simulink model "qp_torq_allocator_base"  (R2024b)
settings: Solver=VariableStepAuto  StartTime=0.0  StopTime=10.0  FixedStep=0.004  RelTol=1e-3
settings Model: Creator=lukec  LastModifiedBy=lukec
settings SolverCC: ZeroCrossControl=DisableAll
settings OptimizationCC: DefaultParameterBehavior=Inlined  EnhancedBackFolding=on  PassReuseOutputArgsAs=Individual arguments  ZeroExternalMemoryAtStartup=off  ZeroInternalMemoryAtStartup=off  OptimizeBlockOrder=speed  DifferentSizesBufferReuse=on  OptimizationCustomize=off  EfficientTunableParamExpr=on
settings DebuggingCC: ParameterTunabilityLossMsg=error
settings HardwareCC: ProdBitPerPointer=32  ProdBitPerSizeT=32  ProdBitPerPtrDiffT=32  ProdLargestAtomicInteger=Long  ProdLargestAtomicFloat=Double  ProdWordSize=32  ProdHWDeviceType=ARM Compatible->ARM Cortex-M
settings SFSimCC: MATLABDynamicMemAlloc=off
settings RTWCC: Description=Embedded Coder  SystemTargetFile=ert.tlc  GenCodeOnly=on  PackageGeneratedCodeAndArtifacts=on  TemplateMakefile=ert_default_tmf  Toolchain=CMake  TargetLang=C++  HalideCodeGeneration=on
settings CodeAppCC: ForceParamTrailComments=on  IgnoreCustomStorageClasses=off  MaxIdLength=255  OperatorAnnotations=on  SimulinkDataObjDesc=on  SFDataObjDesc=on  InsertBlockDesc=on
settings ERTTargetCC: TargetLangStandard=C++17 (ISO)  CodeInterfacePackaging=C++ class  RootIOFormat=Structure reference  ERTCustomFileTemplate=example_file_process.tlc  ArrayContainerType=std::array

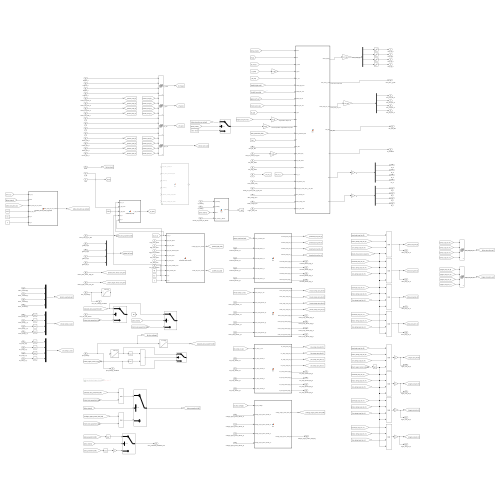
[thumbnail: Simulink's stored preview of the top-level diagram]
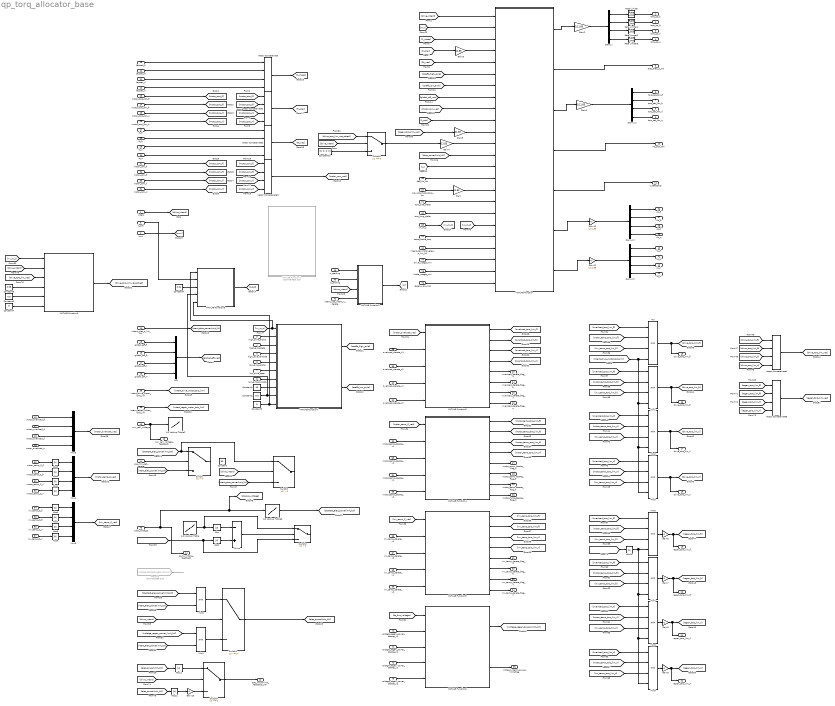
== system qp_torq_allocator_base ==
  intent : Inport
  mux : Inport  Port=2
  high_axle_alpha : Inport  Port=3
  high_axle_beta : Inport  Port=4
  high_axle_lambda : Inport  Port=5
  low_axle_alpha : Inport  Port=6
  low_axle_beta : Inport  Port=7
  low_axle_lambda : Inport  Port=8
  k_opt : Inport  Port=9
  intent_elec_p_lim_kW : Inport  Port=10
  torq_side_delta : Inport  Port=11
  torq_long_delta : Inport  Port=12
  w_starting : Inport  Port=13
  coast_brake_torq : Inport  Port=14
  global_eff_fl : Inport  Port=15
  global_eff_fr : Inport  Port=16
  global_eff_rl : Inport  Port=17
  global_eff_rr : Inport  Port=18
  kappas_fl : Inport  Port=19
  kappas_fr : Inport  Port=20
  kappas_rl : Inport  Port=21
  kappas_rr : Inport  Port=22
  motor_torq_Nm_fl : Inport  Port=23
  motor_torq_Nm_fr : Inport  Port=24
  motor_torq_Nm_rl : Inport  Port=25
  motor_torq_Nm_rr : Inport  Port=26
  fz_fl : Inport  Port=27
  fz_fr : Inport  Port=28
  fz_rl : Inport  Port=29
  fz_rr : Inport  Port=30
  motor_rpm_fl : Inport  Port=31
  motor_rpm_fr : Inport  Port=32
  motor_rpm_rl : Inport  Port=33
  motor_rpm_rr : Inport  Port=34
  vx_m_s : Inport  Port=35
  des_Mz_Nm : Inport  Port=36
  max_tot_motor_torq_Nm : Inport  Port=37
  intent_drive_motor_torq_lim : Inport  Port=38
  intent_regen_motor_torq_lim : Inport  Port=39
  w_ending : Inport  Port=40
  intent_per_motor_elec_p_lim_kW : Inport  Port=41
  intent_use_intent_w_derate : Inport  Port=42  OutDataTypeStr=boolean
  min_cell_voltage : Inport  Port=43
  use_min_cell_derate : Inport  Port=44  OutDataTypeStr=boolean
  pack_voltage : Inport  Port=45
  motor_overload_fl : Inport  Port=46
  motor_overload_fr : Inport  Port=47
  motor_overload_rl : Inport  Port=48
  motor_overload_rr : Inport  Port=49
  motor_temp_C_fl : Inport  Port=50
  motor_temp_C_fr : Inport  Port=51
  motor_temp_C_rl : Inport  Port=52
  motor_temp_C_rr : Inport  Port=53
  inv_temp_C_fl : Inport  Port=54
  inv_temp_C_fr : Inport  Port=55
  inv_temp_C_rl : Inport  Port=56
  inv_temp_C_rr : Inport  Port=57
  overload_derate_x1 : Inport  Port=58
  overload_derate_x2 : Inport  Port=59
  overload_derate_y1 : Inport  Port=60
  overload_derate_y2 : Inport  Port=61
  motor_temp_derate_x1 : Inport  Port=62
  motor_temp_derate_x2 : Inport  Port=63
  motor_temp_derate_y1 : Inport  Port=64
  motor_temp_derate_y2 : Inport  Port=65
  inv_temp_derate_x1 : Inport  Port=66
  inv_temp_derate_x2 : Inport  Port=67
  inv_temp_derate_y1 : Inport  Port=68
  inv_temp_derate_y2 : Inport  Port=69
  voltage_regen_power_derate_x1 : Inport  Port=70
  voltage_regen_power_derate_x2 : Inport  Port=71
  voltage_regen_power_derate_y1 : Inport  Port=72
  voltage_regen_power_derate_y2 : Inport  Port=73
  drive_usage_min : Inport  Port=74
  brake_usage_min : Inport  Port=75
  regen_yaw_max : Inport  Port=76
  1-D Lookup Table : Lookup_n-D  NumberOfTableDimensions=1  BreakpointsForDimension1=[520 530]  Table=[-21 -2]  ExtrapMethod=Clip  UseLastTableValue=on  InternalRulePriority=Speed  RndMeth=Simplest
  1-D Lookup Table2 : Lookup_n-D  NumberOfTableDimensions=1  BreakpointsForDimension1=flip([3.5 3.3 3.15])  Table=flip([78 60 20])  ExtrapMethod=Clip  UseLastTableValue=on  InternalRulePriority=Speed  RndMeth=Simplest
  1-D Lookup Table3 : Lookup_n-D  NumberOfTableDimensions=1  BreakpointsForDimension1=flip([455 445 430])  Table=flip([80 65 40])  ExtrapMethod=Clip  UseLastTableValue=on  InternalRulePriority=Speed  RndMeth=Simplest
  Abs{,1..12} (13 alike) : Abs  SaturateOnIntegerOverflow=off
  Constant : Constant  Value=80
  Constant1 : Constant  Value=40
  Constant10 : Constant  Value=[0; 0; 0; 0]
  Constant2 : Constant  Value=0.5
  Constant3 : Constant  Value=5
  Constant4 : Constant  Value=0.04
  Constant5 : Constant  Value=0.05
  Constant6 : Constant  Value=0.5
  Constant7 : Constant  Value=5
  Demux{,1..3} (4 alike) : Demux
  From10 : From  Commented=on  GotoTag=voltage_derated_regen_torq_lim
  Gain{,3..5} (4 alike) : Gain  Gain=11.83
  Gain{1..2,11..12} (4 alike) : Gain  Gain=1/11.83
  Gain{6..10} (5 alike) : Gain  Gain=-1
  MATLAB Function : MATLAB Function  TreatAsAtomicUnit=on
  MATLAB Function1 : MATLAB Function  Commented=on  TreatAsAtomicUnit=on
  MATLAB Function2 : MATLAB Function  TreatAsAtomicUnit=on
  MATLAB Function3 : MATLAB Function  TreatAsAtomicUnit=on
  MATLAB Function4 : MATLAB Function  TreatAsAtomicUnit=on
  MATLAB Function5 : MATLAB Function  TreatAsAtomicUnit=on
  MATLAB Function6 : MATLAB Function  TreatAsAtomicUnit=on
  MATLAB Function7 : MATLAB Function  TreatAsAtomicUnit=on
  MATLAB Function8 : MATLAB Function  TreatAsAtomicUnit=on
  MATLAB Function9 : MATLAB Function  TreatAsAtomicUnit=on
  Min{,1..3,6..9} (8 alike) : MinMax  Inputs=4
  Min4 : MinMax  Inputs=2
  Min5 : MinMax  Inputs=2
  Minus : Sum  Inputs=-+
  Mux{,3..5} (4 alike) : Mux
  Rate Limiter{,1..3} (4 alike) : RateLimiter  RisingSlewLimit=210  FallingSlewLimit=-210  SampleTimeMode=inherited
  Switch : Switch  Criteria=u2 > Threshold  SaturateOnIntegerOverflow=off  InputSameDT=off
  Switch1 : Switch  Criteria=u2 > Threshold  SaturateOnIntegerOverflow=off  InputSameDT=off
  Switch2 : Switch  Criteria=u2 > Threshold  SaturateOnIntegerOverflow=off  InputSameDT=off
  Switch3 : Switch  SaturateOnIntegerOverflow=off  InputSameDT=off
  Switch4 : Switch  SaturateOnIntegerOverflow=off  InputSameDT=off
  Switch5 : Switch  SaturateOnIntegerOverflow=off  InputSameDT=off
  Vector Concatenate{,1..5} (6 alike) : Concatenate  NumInputs=4  Mode=Multidimensional array
  torq_qp_fl : Outport
  torq_qp_fr : Outport  Port=2
  torq_qp_rl : Outport  Port=3
  torq_qp_rr : Outport  Port=4
  elec_theo_p_kW : Outport  Port=5
  torq_sat_Nm_fl : Outport  Port=6
  torq_sat_Nm_fr : Outport  Port=7
  torq_sat_Nm_rl : Outport  Port=8
  torq_sat_Nm_rr : Outport  Port=9
  Mz_add_Nm : Outport  Port=10
  w_feedback : Outport  Port=11
  elec_powerlimit_feedback_kW : Outport  Port=12
  min_cell_voltage_feedback : Outport  Port=13
  pack_voltage_feedback : Outport  Port=14
  drive_torq_lim_fl : Outport  Port=15
  drive_torq_lim_fr : Outport  Port=16
  drive_torq_lim_rl : Outport  Port=17
  drive_torq_lim_rr : Outport  Port=18
  regen_torq_lim_fl : Outport  Port=19
  regen_torq_lim_fr : Outport  Port=20
  regen_torq_lim_rl : Outport  Port=21
  regen_torq_lim_rr : Outport  Port=22
  overload_derate_flag_fl : Outport  Port=23
  overload_derate_flag_fr : Outport  Port=24
  overload_derate_flag_rl : Outport  Port=25
  overload_derate_flag_rr : Outport  Port=26
  motor_temp_derate_flag_fl : Outport  Port=27
  motor_temp_derate_flag_fr : Outport  Port=28
  motor_temp_derate_flag_rl : Outport  Port=29
  motor_temp_derate_flag_rr : Outport  Port=30
  inv_temp_derate_flag_fl : Outport  Port=31
  inv_temp_derate_flag_fr : Outport  Port=32
  inv_temp_derate_flag_rl : Outport  Port=33
  inv_temp_derate_flag_rr : Outport  Port=34
  voltage_regen_power_limit_flag : Outport  Port=35
  ub_fl : Outport  Port=36
  ub_fr : Outport  Port=37
  ub_rl : Outport  Port=38
  ub_rr : Outport  Port=39
  lb_fl : Outport  Port=40
  lb_fr : Outport  Port=41
  lb_rl : Outport  Port=42
  lb_rr : Outport  Port=43
  wires:
  [Fz_vec] -> MATLAB Function/5(Fz_vec)
  [motor_torq_fl] -> Vector Concatenate1/1
  fz_rl/1 -> Vector Concatenate2/3
  motor_rpm_fl/1 -> [motor_rpm_fl]
  Mux/1 -> [global_eff_vec]
  [motor_torq_rl] -> Vector Concatenate1/3
  Vector Concatenate3/1 -> [motor_rpm_vec]  "rpm_vec"
  Constant10/1 -> Switch3/3
  motor_rpm_rr/1 -> [motor_rpm_rr]
  des_Mz_Nm/1 -> MATLAB Function/15(Mz_des)
  fz_fl/1 -> Vector Concatenate2/1
  low_axle_beta/1 -> MATLAB Function7/6(low_axle_beta)
  Gain5/1 -> MATLAB Function/11("lb ")  "Single Wheel Torque LB"
  fz_rr/1 -> Vector Concatenate2/4
  Gain/1 -> MATLAB Function/16(tot_wheel_torq)
  motor_torq_Nm_rr/1 -> [motor_torq_rr]
  motor_rpm_rl/1 -> [motor_rpm_rl]
  [drive_intent] -> Switch3/2
  MATLAB Function/1(wheel_torque) -> Gain2/1
  MATLAB Function/2(elec_theo_p_kW) -> elec_theo_p_kW/1  "Theo. Elec. Power kW"
  fz_fr/1 -> Vector Concatenate2/2
  [motor_torq_rr] -> Vector Concatenate1/4
  motor_torq_Nm_fr/1 -> [motor_torq_fr]
  [motor_torq_fr] -> Vector Concatenate1/2
  [K_meas] -> MATLAB Function/3(K_meas)
  Vector Concatenate/1 -> [K_meas]  "K_meas"
  high_axle_lambda/1 -> MATLAB Function7/4(high_axle_lambda_base)
  [regen_torq_lim_vec] -> Gain5/1
  global_eff_fl/1 -> Mux/1
  MATLAB Function/3(wheel_torq_sat_vec) -> Gain1/1  "wheel_torq_sat_vec"
  max_tot_motor_torq_Nm/1 -> Gain/1
  Gain4/1 -> MATLAB Function/12("ub ")  "Intent Dependent Single Wheel Torque UB"
  [elec_powerlimit_kW] -> MATLAB Function/13(elec_powerlimit_kW)
  kappas_rr/1 -> Vector Concatenate/4
  intent_elec_p_lim_kW/1 -> [intent_elec_powerlimit_kW]
  high_axle_alpha/1 -> MATLAB Function7/2(high_axle_alpha)
  kappas_fl/1 -> Vector Concatenate/1
  low_axle_alpha/1 -> MATLAB Function7/5(low_axle_alpha)
  torq_side_delta/1 -> MATLAB Function/17(torq_side_delta)
  [drive_torq_lim_vec_sched] -> Switch3/1
  Vector Concatenate2/1 -> [Fz_vec]  "Fz_vec"
  [motor_rpm_fl] -> Vector Concatenate3/1
  kappas_fr/1 -> Vector Concatenate/2
  motor_rpm_fr/1 -> [motor_rpm_fr]
  motor_torq_Nm_rl/1 -> [motor_torq_rl]
  motor_torq_Nm_fl/1 -> [motor_torq_fl]
  [motor_rpm_fr] -> Vector Concatenate3/2
  [motor_rpm_vec] -> MATLAB Function/9(motor_rpm_vec)
  low_axle_lambda/1 -> MATLAB Function7/7(low_axle_lambda_base)
  high_axle_beta/1 -> MATLAB Function7/3(high_axle_beta)
  Gain2/1 -> Demux/1  "motor_torque_qp"
  [coeffs_low_axle] -> MATLAB Function/7(coeffs_low_axle)
  [coeffs_high_axle] -> MATLAB Function/6(coeffs_high_axle)
  [k_opt] -> MATLAB Function/10(K_opt)
  Vector Concatenate1/1 -> [T_prev]  "T_prev"
  [motor_rpm_rl] -> Vector Concatenate3/3
  kappas_rl/1 -> Vector Concatenate/3
  [global_eff_vec] -> MATLAB Function/8(global_eff_vec)
  global_eff_rl/1 -> Mux/3
  coast_brake_torq/1 -> MATLAB Function/20(coast_brake_torq)
  [drive_intent] -> MATLAB Function/1(intent)
  intent/1 -> [drive_intent]
  [motor_rpm_rr] -> Vector Concatenate3/4
  global_eff_fr/1 -> Mux/2
  Gain3/1 -> MATLAB Function/4(T_prev)
  [T_prev] -> Gain3/1
  mux/1 -> [mux]
  global_eff_rr/1 -> Mux/4
  intent_drive_motor_torq_lim/1 -> [intent_drive_motor_torq_lim]
  intent_regen_motor_torq_lim/1 -> [intent_regen_motor_torq_lim]
  torq_long_delta/1 -> MATLAB Function/18(torq_long_delta)
  Gain1/1 -> Demux1/1
  Demux1/1 -> torq_sat_Nm_fl/1
  Demux1/2 -> torq_sat_Nm_fr/1
  Demux1/3 -> torq_sat_Nm_rl/1
  Demux1/4 -> torq_sat_Nm_rr/1
  MATLAB Function/4(Mz_add) -> Mz_add_Nm/1  "Mz_add"
  MATLAB Function/5(w) -> w_feedback/1
  intent_per_motor_elec_p_lim_kW/1 -> MATLAB Function/21(intent_per_motor_elec_p_lim_kW)
  [mux] -> MATLAB Function/2(mux)
  w_starting/1 -> MATLAB Function2/1(w_starting)
  [drive_intent] -> MATLAB Function2/3(intent)
  w_ending/1 -> MATLAB Function2/2(w_ending)
  intent_use_intent_w_derate/1 -> MATLAB Function2/4(use_intent_w_derate)
  MATLAB Function2/1(w_derate) -> [w]
  [w] -> MATLAB Function/14("w ")
  use_min_cell_derate/1 -> Switch/2
  [derated_elec_powerlimit_kW] -> Switch1/1, Switch/1
  [intent_elec_powerlimit_kW] -> Switch/3
  [drive_intent] -> Switch1/2
  [intent_elec_powerlimit_kW] -> Switch1/3
  pack_voltage/1 -> [dc_bus_voltage], 1-D Lookup Table3/1, pack_voltage_feedback/1
  1-D Lookup Table/1 -> Switch2/1, Abs/1
  [intent_regen_motor_torq_lim] -> Switch2/3, Abs1/1
  Abs/1 -> Minus/1
  Abs1/1 -> Minus/2
  Minus/1 -> Switch2/2
  min_cell_voltage/1 -> 1-D Lookup Table2/1, min_cell_voltage_feedback/1
  From10/1 -> ?
  1-D Lookup Table3/1 -> [derated_elec_powerlimit_kW]
  motor_overload_fl/1 -> Mux3/1
  motor_overload_fr/1 -> Mux3/2
  motor_overload_rl/1 -> Mux3/3
  motor_overload_rr/1 -> Mux3/4
  Mux3/1 -> [motor_overload_vec]
  motor_temp_C_fl/1 -> Abs2/1
  motor_temp_C_fr/1 -> Abs3/1
  motor_temp_C_rl/1 -> Abs4/1
  motor_temp_C_rr/1 -> Abs5/1
  Mux4/1 -> [motor_temp_C_vec]
  inv_temp_C_fl/1 -> Abs6/1
  inv_temp_C_fr/1 -> Abs7/1
  inv_temp_C_rl/1 -> Abs8/1
  inv_temp_C_rr/1 -> Abs9/1
  Mux5/1 -> [inv_temp_C_vec]
  [motor_overload_vec] -> MATLAB Function3/1(motor_overload_vec)
  overload_derate_x1/1 -> MATLAB Function3/2(overload_derate_x1)
  overload_derate_x2/1 -> MATLAB Function3/3(overload_derate_x2)
  overload_derate_y1/1 -> MATLAB Function3/4(overload_derate_y1)
  overload_derate_y2/1 -> MATLAB Function3/5(overload_derate_y2)
  [motor_temp_C_vec] -> MATLAB Function4/1(motor_temp_C_vec)
  motor_temp_derate_x1/1 -> MATLAB Function4/2(motor_temp_derate_x1)
  motor_temp_derate_x2/1 -> MATLAB Function4/3(motor_temp_derate_x2)
  motor_temp_derate_y1/1 -> MATLAB Function4/4(motor_temp_derate_y1)
  motor_temp_derate_y2/1 -> MATLAB Function4/5(motor_temp_derate_y2)
  Abs2/1 -> Mux4/1
  Abs3/1 -> Mux4/2
  Abs4/1 -> Mux4/3
  Abs5/1 -> Mux4/4
  Abs6/1 -> Mux5/1
  Abs7/1 -> Mux5/2
  Abs8/1 -> Mux5/3
  Abs9/1 -> Mux5/4
  [inv_temp_C_vec] -> MATLAB Function5/1(inv_temp_C_vec)
  inv_temp_derate_x1/1 -> MATLAB Function5/2(inv_temp_derate_x1)
  inv_temp_derate_x2/1 -> MATLAB Function5/3(inv_temp_derate_x2)
  inv_temp_derate_y1/1 -> MATLAB Function5/4(inv_temp_derate_y1)
  inv_temp_derate_y2/1 -> MATLAB Function5/5(inv_temp_derate_y2)
  MATLAB Function3/1(overload_torq_lim_fl) -> [overload_torq_lim_fl]
  MATLAB Function3/2(overload_torq_lim_fr) -> [overload_torq_lim_fr]
  MATLAB Function3/3(overload_torq_lim_rl) -> [overload_torq_lim_rl]
  MATLAB Function3/4(overload_torq_lim_rr) -> [overload_torq_lim_rr]
  MATLAB Function4/1(motor_temp_torq_lim_fl) -> [motor_temp_torq_lim_fl]
  MATLAB Function4/2(motor_temp_torq_lim_fr) -> [motor_temp_torq_lim_fr]
  MATLAB Function4/3(motor_temp_torq_lim_rl) -> [motor_temp_torq_lim_rl]
  MATLAB Function4/4(motor_temp_torq_lim_rr) -> [motor_temp_torq_lim_rr]
  MATLAB Function5/1(inv_temp_torq_lim_fl) -> [inv_temp_torq_lim_fl]
  MATLAB Function5/2(inv_temp_torq_lim_fr) -> [inv_temp_torq_lim_fr]
  MATLAB Function5/3(inv_temp_torq_lim_rl) -> [inv_temp_torq_lim_rl]
  MATLAB Function5/4(inv_temp_torq_lim_rr) -> [inv_temp_torq_lim_rr]
  [motor_temp_torq_lim_fl] -> Min/2
  [inv_temp_torq_lim_fl] -> Min/3
  [overload_torq_lim_fl] -> Min/1
  [overload_torq_lim_fr] -> Min1/1
  [inv_temp_torq_lim_fr] -> Min1/3
  [motor_temp_torq_lim_fr] -> Min1/2
  [motor_temp_torq_lim_rr] -> Min3/2
  [inv_temp_torq_lim_rr] -> Min3/3
  [overload_torq_lim_rr] -> Min3/1
  [overload_torq_lim_rl] -> Min2/1
  [inv_temp_torq_lim_rl] -> Min2/3
  [motor_temp_torq_lim_rl] -> Min2/2
  Min/1 -> drive_torq_lim_fl/1, [drive_torq_lim_fl]
  Min1/1 -> drive_torq_lim_fr/1, [drive_torq_lim_fr]
  Min2/1 -> drive_torq_lim_rl/1, [drive_torq_lim_rl]
  Min3/1 -> drive_torq_lim_rr/1, [drive_torq_lim_rr]
  [intent_drive_motor_torq_lim] -> Min2/4, Min3/4, Min1/4, Min/4
  [drive_torq_lim_fl] -> Vector Concatenate4/1
  [drive_torq_lim_fr] -> Vector Concatenate4/2
  [drive_torq_lim_rl] -> Vector Concatenate4/3
  [drive_torq_lim_rr] -> Vector Concatenate4/4
  Vector Concatenate4/1 -> [drive_torq_lim_vec]  "drive_torq_lim_vec"
  [dc_bus_voltage] -> MATLAB Function6/1(dc_bus_voltage)
  voltage_regen_power_derate_x1/1 -> MATLAB Function6/2(voltage_regen_power_derate_x1)
  voltage_regen_power_derate_x2/1 -> MATLAB Function6/3(voltage_regen_power_derate_x2)
  voltage_regen_power_derate_y1/1 -> MATLAB Function6/4(voltage_regen_power_derate_y1)
  voltage_regen_power_derate_y2/1 -> MATLAB Function6/5(voltage_regen_power_derate_y2)
  MATLAB Function6/1(voltage_regen_power_limit_kW) -> [voltage_regen_power_limit_kW]
  [drive_intent] -> Switch4/2
  [voltage_regen_power_limit_kW] -> Min4/1
  [intent_elec_powerlimit_kW] -> Min4/2
  [derated_elec_powerlimit_kW] -> Min5/1
  [intent_elec_powerlimit_kW] -> Min5/2
  Min5/1 -> Switch4/1
  Min4/1 -> Switch4/3
  Switch4/1 -> [elec_powerlimit_kW]
  [intent_regen_motor_torq_lim] -> Abs10/1
  Min9/1 -> Gain9/1
  Min8/1 -> Gain8/1
  Min7/1 -> Gain7/1
  Min6/1 -> Gain6/1
  [motor_temp_torq_lim_rl] -> Min8/2
  [inv_temp_torq_lim_rl] -> Min8/3
  [overload_torq_lim_rl] -> Min8/1
  [overload_torq_lim_rr] -> Min9/1
  [inv_temp_torq_lim_rr] -> Min9/3
  [motor_temp_torq_lim_rr] -> Min9/2
  [motor_temp_torq_lim_fr] -> Min7/2
  [inv_temp_torq_lim_fr] -> Min7/3
  [overload_torq_lim_fr] -> Min7/1
  [overload_torq_lim_fl] -> Min6/1
  [inv_temp_torq_lim_fl] -> Min6/3
  [motor_temp_torq_lim_fl] -> Min6/2
  Abs10/1 -> Min6/4, Min7/4, Min9/4, Min8/4
  Gain6/1 -> regen_torq_lim_fl/1, [regen_torq_lim_fl]
  Gain7/1 -> regen_torq_lim_fr/1, [regen_torq_lim_fr]
  Gain8/1 -> regen_torq_lim_rl/1, [regen_torq_lim_rl]
  Gain9/1 -> regen_torq_lim_rr/1, [regen_torq_lim_rr]
  Vector Concatenate5/1 -> [regen_torq_lim_vec]  "regen_torq_lim_vec"
  [regen_torq_lim_rr] -> Vector Concatenate5/4
  [regen_torq_lim_rl] -> Vector Concatenate5/3
  [regen_torq_lim_fr] -> Vector Concatenate5/2
  [regen_torq_lim_fl] -> Vector Concatenate5/1
  MATLAB Function3/5(overload_derate_flag_fl) -> overload_derate_flag_fl/1
  MATLAB Function3/6(overload_derate_flag_fr) -> overload_derate_flag_fr/1
  MATLAB Function3/7(overload_derate_flag_rl) -> overload_derate_flag_rl/1
  MATLAB Function3/8(overload_derate_flag_rr) -> overload_derate_flag_rr/1
  MATLAB Function4/5(motor_temp_derate_flag_fl) -> motor_temp_derate_flag_fl/1
  MATLAB Function4/6(motor_temp_derate_flag_fr) -> motor_temp_derate_flag_fr/1
  MATLAB Function4/7(motor_temp_derate_flag_rl) -> motor_temp_derate_flag_rl/1
  MATLAB Function4/8(motor_temp_derate_flag_rr) -> motor_temp_derate_flag_rr/1
  MATLAB Function5/5(inv_temp_derate_flag_fl) -> inv_temp_derate_flag_fl/1
  MATLAB Function5/6(inv_temp_derate_flag_fr) -> inv_temp_derate_flag_fr/1
  MATLAB Function5/7(inv_temp_derate_flag_rl) -> inv_temp_derate_flag_rl/1
  MATLAB Function5/8(inv_temp_derate_flag_rr) -> inv_temp_derate_flag_rr/1
  MATLAB Function6/2(voltage_regen_power_limit_flag) -> voltage_regen_power_limit_flag/1
  [drive_intent] -> Switch5/2
  [elec_powerlimit_kW] -> Abs11/1
  [elec_powerlimit_kW] -> Abs12/1
  Abs11/1 -> Switch5/1
  Abs12/1 -> Gain10/1
  Gain10/1 -> Switch5/3
  Switch5/1 -> elec_powerlimit_feedback_kW/1
  Switch3/1 -> Gain4/1
  MATLAB Function/7(lb) -> Gain11/1
  MATLAB Function/6(ub) -> Gain12/1
  Gain12/1 -> Demux2/1  "ub"
  Demux2/1 -> ub_fl/1
  Demux2/2 -> ub_fr/1
  Demux2/3 -> ub_rl/1
  Demux2/4 -> ub_rr/1
  Demux3/4 -> lb_rr/1
  Demux3/3 -> lb_rl/1
  Demux3/2 -> lb_fr/1
  Gain11/1 -> Demux3/1  "ub"
  Demux3/1 -> lb_fl/1
  drive_usage_min/1 -> MATLAB Function/22(drive_usage_min)
  brake_usage_min/1 -> MATLAB Function/23(brake_usage_min)
  Demux/1 -> Rate Limiter/1
  Demux/2 -> Rate Limiter1/1
  Demux/3 -> Rate Limiter2/1
  Demux/4 -> Rate Limiter3/1
  Rate Limiter/1 -> torq_qp_fl/1
  Rate Limiter1/1 -> torq_qp_fr/1
  Rate Limiter2/1 -> torq_qp_rl/1
  Rate Limiter3/1 -> torq_qp_rr/1
  vx_m_s/1 -> [vx_m_s]
  [vx_m_s] -> MATLAB Function/19(vx_m_s)
  [vx_m_s] -> MATLAB Function8/1(vx_m_s), MATLAB Function7/1(vx_m_s)
  Constant1/1 -> MATLAB Function7/8(delta_lambda_low)
  Constant2/1 -> MATLAB Function8/4(vx_lo), MATLAB Function7/9(vx_lo)
  Constant3/1 -> MATLAB Function8/5(vx_hi), MATLAB Function7/10(vx_hi)
  MATLAB Function7/1(coeffs_high_axle_sched) -> [coeffs_high_axle]
  MATLAB Function7/2(coeffs_low_axle_sched) -> [coeffs_low_axle]
  Constant4/1 -> MATLAB Function8/3(k_opt_low)
  k_opt/1 -> MATLAB Function8/2(k_opt_nom)
  MATLAB Function8/1(k_opt_sched) -> [k_opt]
  [drive_torq_lim_vec] -> MATLAB Function9/3(drive_torq_lim_vec_base)
  Constant5/1 -> MATLAB Function9/4(low_cap_min)
  Constant6/1 -> MATLAB Function9/5(vx_lo)
  Constant7/1 -> MATLAB Function9/6(vx_hi)
  [drive_intent] -> MATLAB Function9/2(intent)
  [vx_m_s] -> MATLAB Function9/1(vx_m_s)
  MATLAB Function9/1(drive_torq_lim_vec_sched) -> [drive_torq_lim_vec_sched]
  regen_yaw_max/1 -> MATLAB Function/24(regen_yaw_max)

== matlab function qp_torq_allocator_base/MATLAB Function4 ==
  data: motor_temp_C_vec input; motor_temp_torq_lim_fl output; motor_temp_derate_x1 input; motor_temp_derate_x2 input; motor_temp_derate_y1 input; motor_temp_derate_y2 input; motor_temp_torq_lim_fr output; motor_temp_torq_lim_rl output; motor_temp_torq_lim_rr output; motor_temp_derate_flag_fl output; motor_temp_derate_flag_fr output; motor_temp_derate_flag_rl output; motor_temp_derate_flag_rr output
function  [motor_temp_torq_lim_fl, motor_temp_torq_lim_fr, motor_temp_torq_lim_rl, motor_temp_torq_lim_rr, motor_temp_derate_flag_fl, motor_temp_derate_flag_fr, motor_temp_derate_flag_rl, motor_temp_derate_flag_rr] = fcn(motor_temp_C_vec, motor_temp_derate_x1, motor_temp_derate_x2, motor_temp_derate_y1, motor_temp_derate_y2)

overload_torq_lim = zeros(4, 1);
overload_derate_flag = zeros(4, 1);

for i = 1:length(motor_temp_C_vec)
    if motor_temp_C_vec(i) > motor_temp_derate_x2
        motor_temp_C_vec(i) = motor_temp_derate_x2;
    end

    if motor_temp_C_vec(i) < motor_temp_derate_x1
        motor_temp_C_vec(i) = motor_temp_derate_x1;
    end

    overload_torq_lim(i) = interp1([motor_temp_derate_x1, motor_temp_derate_x2], [motor_temp_derate_y1, motor_temp_derate_y2], motor_temp_C_vec(i));
    
    if overload_torq_lim(i) < motor_temp_derate_y1
        overload_derate_flag(i) = 1;
    end
end

motor_temp_torq_lim_fl = overload_torq_lim(1);
motor_temp_torq_lim_fr = overload_torq_lim(2);
motor_temp_torq_lim_rl = overload_torq_lim(3);
motor_temp_torq_lim_rr = overload_torq_lim(4);

motor_temp_derate_flag_fl = overload_derate_flag(1);
motor_temp_derate_flag_fr = overload_derate_flag(2);
motor_temp_derate_flag_rl = overload_derate_flag(3);
motor_temp_derate_flag_rr = overload_derate_flag(4);

== matlab function qp_torq_allocator_base/MATLAB Function5 ==
  data: inv_temp_C_vec input; inv_temp_torq_lim_fl output; inv_temp_derate_x1 input; inv_temp_derate_x2 input; inv_temp_derate_y1 input; inv_temp_derate_y2 input; inv_temp_torq_lim_fr output; inv_temp_torq_lim_rl output; inv_temp_torq_lim_rr output; inv_temp_derate_flag_fl output; inv_temp_derate_flag_fr output; inv_temp_derate_flag_rl output; inv_temp_derate_flag_rr output
function  [inv_temp_torq_lim_fl, inv_temp_torq_lim_fr, inv_temp_torq_lim_rl, inv_temp_torq_lim_rr, inv_temp_derate_flag_fl, inv_temp_derate_flag_fr, inv_temp_derate_flag_rl, inv_temp_derate_flag_rr] = fcn(inv_temp_C_vec, inv_temp_derate_x1, inv_temp_derate_x2, inv_temp_derate_y1, inv_temp_derate_y2)

overload_torq_lim = zeros(4, 1);
overload_derate_flag = zeros(4, 1);

for i = 1:length(inv_temp_C_vec)
    if inv_temp_C_vec(i) > inv_temp_derate_x2
        inv_temp_C_vec(i) = inv_temp_derate_x2;
    end

    if inv_temp_C_vec(i) < inv_temp_derate_x1
        inv_temp_C_vec(i) = inv_temp_derate_x1;
    end

    overload_torq_lim(i) = interp1([inv_temp_derate_x1, inv_temp_derate_x2], [inv_temp_derate_y1, inv_temp_derate_y2], inv_temp_C_vec(i));
    
    if overload_torq_lim(i) < inv_temp_derate_y1
        overload_derate_flag(i) = 1;
    end
end

inv_temp_torq_lim_fl = overload_torq_lim(1);
inv_temp_torq_lim_fr = overload_torq_lim(2);
inv_temp_torq_lim_rl = overload_torq_lim(3);
inv_temp_torq_lim_rr = overload_torq_lim(4);

inv_temp_derate_flag_fl = overload_derate_flag(1);
inv_temp_derate_flag_fr = overload_derate_flag(2);
inv_temp_derate_flag_rl = overload_derate_flag(3);
inv_temp_derate_flag_rr = overload_derate_flag(4);

== matlab function qp_torq_allocator_base/MATLAB Function6 ==
  data: dc_bus_voltage input; voltage_regen_power_limit_kW output; voltage_regen_power_derate_x1 input; voltage_regen_power_derate_x2 input; voltage_regen_power_derate_y1 input; voltage_regen_power_derate_y2 input; voltage_regen_power_limit_flag output
function [voltage_regen_power_limit_kW, voltage_regen_power_limit_flag] = fcn(dc_bus_voltage, voltage_regen_power_derate_x1, voltage_regen_power_derate_x2, voltage_regen_power_derate_y1, voltage_regen_power_derate_y2)

voltage_regen_power_limit_flag = 0;

if dc_bus_voltage < voltage_regen_power_derate_x1
    dc_bus_voltage = voltage_regen_power_derate_x1;
end

if dc_bus_voltage > voltage_regen_power_derate_x2
    dc_bus_voltage = voltage_regen_power_derate_x2;
end

voltage_regen_power_limit_kW = interp1([voltage_regen_power_derate_x1, voltage_regen_power_derate_x2], [voltage_regen_power_derate_y1, voltage_regen_power_derate_y2], dc_bus_voltage);


if voltage_regen_power_limit_kW < voltage_regen_power_derate_y1
    voltage_regen_power_limit_flag = 1;
end

== matlab function qp_torq_allocator_base/MATLAB Function7 ==
  data: vx_m_s input; coeffs_high_axle_sched output; high_axle_alpha input; high_axle_beta input; high_axle_lambda_base input; low_axle_alpha input; low_axle_beta input; low_axle_lambda_base input; delta_lambda_low input; vx_lo input; vx_hi input; coeffs_low_axle_sched output
function [coeffs_high_axle_sched, coeffs_low_axle_sched] = ...
    schedule_axle_coeffs(vx_m_s, ...
    high_axle_alpha, high_axle_beta, high_axle_lambda_base, ...
    low_axle_alpha,  low_axle_beta,  low_axle_lambda_base, ...
    delta_lambda_low, vx_lo, vx_hi)

    s_vx = (vx_m_s - vx_lo) / (vx_hi - vx_lo);
    s_vx = min(max(s_vx, 0), 1);

    lambda_high_sched = high_axle_lambda_base;
    lambda_low_sched  = low_axle_lambda_base + (1 - s_vx) * delta_lambda_low;

    coeffs_high_axle_sched = [high_axle_alpha; high_axle_beta; lambda_high_sched];
    coeffs_low_axle_sched  = [low_axle_alpha;  low_axle_beta;  lambda_low_sched];
end

== matlab function qp_torq_allocator_base/MATLAB Function8 ==
  data: vx_m_s input; k_opt_sched output; k_opt_nom input; k_opt_low input; vx_lo input; vx_hi input
function k_opt_sched = schedule_kopt(vx_m_s, k_opt_nom, k_opt_low, vx_lo, vx_hi)

    s_vx = (vx_m_s - vx_lo) / (vx_hi - vx_lo);
    s_vx = min(max(s_vx, 0), 1);

    k_opt_sched = k_opt_low + s_vx * (k_opt_nom - k_opt_low);
end

== matlab function qp_torq_allocator_base/MATLAB Function9 ==
  data: vx_m_s input; drive_torq_lim_vec_sched output; intent input; drive_torq_lim_vec_base input; low_cap_min input; vx_lo input; vx_hi input
function drive_torq_lim_vec_sched = schedule_drive_limits_highlow( ...
    vx_m_s, intent, drive_torq_lim_vec_base, low_cap_min, vx_lo, vx_hi)

    s_vx = (vx_m_s - vx_lo) / (vx_hi - vx_lo);
    s_vx = min(max(s_vx, 0), 1);

    gamma_low = low_cap_min + (1 - low_cap_min) * s_vx;

    drive_torq_lim_vec_sched = drive_torq_lim_vec_base;

    if intent >= 0
        % accel/coast: low axle = front = FL, FR
        drive_torq_lim_vec_sched(1) = gamma_low * drive_torq_lim_vec_base(1);
        drive_torq_lim_vec_sched(2) = gamma_low * drive_torq_lim_vec_base(2);
    else
        % braking: low axle = rear = RL, RR
        drive_torq_lim_vec_sched(3) = gamma_low * drive_torq_lim_vec_base(3);
        drive_torq_lim_vec_sched(4) = gamma_low * drive_torq_lim_vec_base(4);
    end
end

== matlab function qp_torq_allocator_base/MATLAB Function ==
  data: intent input; mux input; K_meas input; wheel_torque output; T_prev input; Fz_vec input; coeffs_high_axle input; coeffs_low_axle input; global_eff_vec input; motor_rpm_vec input; K_opt input; lb input; ub input; elec_theo_p_kW output; wheel_torq_sat_vec output; elec_powerlimit_kW input; w input; Mz_des input; tot_wheel_torq input; Mz_add output; torq_side_delta input; torq_long_delta input; vx_m_s input; coast_brake_torq input; w output; ub output; intent_per_motor_elec_p_lim_kW input; lb output; drive_usage_min input; brake_usage_min input; regen_yaw_max input
function [wheel_torque, elec_theo_p_kW, wheel_torq_sat_vec, Mz_add, w, ub, lb] = fcn(intent, mux, K_meas, T_prev, Fz_vec, ...
    coeffs_high_axle, coeffs_low_axle, global_eff_vec, motor_rpm_vec, K_opt, lb, ub, elec_powerlimit_kW, w, Mz_des, tot_wheel_torq, ...
    torq_side_delta, torq_long_delta, vx_m_s, coast_brake_torq, intent_per_motor_elec_p_lim_kW, drive_usage_min, brake_usage_min, regen_yaw_max)

    % if w < 0.08
    %     w = 0.08;
    % end

    % drive_usage_bias = 0.8;
    % brake_usage_bias = 0.9;

    % =========================================================================
    % Constants / geometry
    % =========================================================================
    tot_wheel_torq = abs(tot_wheel_torq);

    rpm2rad_s = 0.10472;
    r  = 0.2;       % effective tire radius, an approximation [m]
    ht = 1.2 / 2;   % half-track [m]

    % =========================================================================
    % Interpolation data for longitudinal stiffness approximation C_kappa(Fz)
    % =========================================================================
    Fz_testpoints = [-100	-150	-200	-250	-300	-350	-400	-450	-500	-550	-600	-650	-700	-750	-800	-850	-900	-950	-1000	-1050	-1100	-1150	-1200	-1250	-1300	-1350	-1400	-1450	-1500	-1550	-1600	-1650	-1700	-1750	-1800	-1850	-1900	-1950	-2000] .* -1;
    CK_testpoints = [4993.96037580768	7230.15025002608	9312.63116671493	11255.0952723015	13070.0418608112	14768.7810353328	16361.4690854774	17857.1668314117	19263.9134694458	20588.8097872709	21838.1058844771	23017.2896709141	24131.1733923846	25183.9762444061	26179.4017891894	27120.7094051015	28010.7793914951	28852.1716449660	29647.1780346286	30397.8687505021	31106.1329947657	31773.7144422382	32402.2419235013	32993.2557891554	33548.2304026337	34068.5931861850	34555.7406132517	35011.0515026319	35435.8979267288	35831.6539982093	36199.7027460456	36541.4412318642	36858.2839884342	37151.6647804853	37423.0365888119	37673.8695948128	37905.6467846387	38119.8565869283	38317.9816880605];


    % =========================================================================
    % Build C_kappa vector and wheel saturation torques
    % =========================================================================
    CK_vec = zeros(4, 1);
    wheel_torq_peak_vec = CK_vec;

    for i = 1:4
        
        if Fz_vec(i) < min(Fz_testpoints)
            Fz_vec(i) = min(Fz_testpoints);
        elseif Fz_vec(i) > max(Fz_testpoints)
            Fz_vec(i) = max(Fz_testpoints);
        end

        CK_vec(i) = interp1(Fz_testpoints', CK_testpoints', Fz_vec(i));
        wheel_torq_peak_vec(i) = Fz_vec(i) * mux * r;
    end

    peak_net_wheel_torq = sum(wheel_torq_peak_vec);
    net_fz = sum(Fz_vec);

    if abs(net_fz) < eps
        perc_fz = 0.25 * ones(4,1);
    else
        perc_fz = abs(Fz_vec ./ net_fz);
    end

    wheel_torq_sat_vec = perc_fz .* peak_net_wheel_torq;


    % =========================================================================
    % Select weights / sign conventions based on driver intent
    % =========================================================================
    if intent >= 0

        alpha_vec  = [coeffs_low_axle(1), coeffs_low_axle(1), coeffs_high_axle(1), coeffs_high_axle(1)];
        beta_vec   = [coeffs_low_axle(2), coeffs_low_axle(2), coeffs_high_axle(2), coeffs_high_axle(2)];
        lambda_vec = [coeffs_low_axle(3), coeffs_low_axle(3), coeffs_high_axle(3), coeffs_high_axle(3)];

        % if abs(Mz_des) < 10 && intent == 0
        %     lb = 0 .* 11.83 .* ones(4, 1);
        % elseif abs(Mz_des) > 10 && intent == 0
        %     lb = coast_brake_torq .* 11.83 .* ones(4, 1);
        % else
        %     lb = 0 .* 11.83 .* ones(4, 1);
        % end
        
        if intent == 0
            % Coast case:
            % keep net torque constrained through A_eq*x = 0,
            % but do NOT force each individual wheel torque to zero.
            if abs(Mz_des) < 10
                lb = zeros(4,1);
            else
                lb = coast_brake_torq * 11.83 * ones(4,1);
            end
        else
            lb = (tot_wheel_torq / 4) * drive_usage_min * ones(4,1);
            lb = min(lb, wheel_torq_sat_vec);

            Mz_thresh = 100;
            vx_thresh = 2;

            if intent > 0 && abs(Mz_des) > Mz_thresh && vx_m_s > vx_thresh
                if Mz_des > 0
                    lb(1) = -regen_yaw_max * 11.83;   % FL
                    lb(3) = -regen_yaw_max * 11.83;   % RL
                else
                    lb(2) = -regen_yaw_max * 11.83;   % FR
                    lb(4) = -regen_yaw_max * 11.83;   % RR
                end
            end
        end

        % if intent > 0
        %     % powerlim_tot_wheel_torq = elec_powerlimit_kW .* 1000 / (sum(motor_rpm_vec(i) * rpm2rad_s / global_eff_vec(i)));
        %     lb = tot_wheel_torq ./ 4 .* [(drive_usage_min), (drive_usage_min), (drive_usage_min), (drive_usage_min)]';
        %     lb(1) = min(lb(1), wheel_torq_sat_vec(1));
        %     lb(2) = min(lb(2), wheel_torq_sat_vec(2));
        %     lb(3) = min(lb(3), wheel_torq_sat_vec(3));
        %     lb(4) = min(lb(4), wheel_torq_sat_vec(4));
        % end

    else
        
        alpha_vec  = [coeffs_high_axle(1), coeffs_high_axle(1), coeffs_low_axle(1), coeffs_low_axle(1)];
        beta_vec   = [coeffs_high_axle(2), coeffs_high_axle(2), coeffs_low_axle(2), coeffs_low_axle(2)];
        lambda_vec = [coeffs_high_axle(3), coeffs_high_axle(3), coeffs_low_axle(3), coeffs_low_axle(3)];

        % Braking sign convention
        alpha_vec = abs(alpha_vec) .* -1;
        K_opt     = abs(K_opt) * -1;
       

        ub = -(tot_wheel_torq / 4) * brake_usage_min * ones(4,1);
        ub = max(ub, -wheel_torq_sat_vec);
        % ub = tot_wheel_torq ./ 4 .* [(brake_usage_min), (brake_usage_min), (brake_usage_min), (brake_usage_min)]' .* -1;
        % ub(1) = max(ub(1), -wheel_torq_sat_vec(1));
        % ub(2) = max(ub(2), -wheel_torq_sat_vec(2));
        % ub(3) = max(ub(3), -wheel_torq_sat_vec(3));
        % ub(4) = max(ub(4), -wheel_torq_sat_vec(4));
    end

    % =========================================================================
    % Build f and H
    % =========================================================================
    ele = zeros(4, 1);
    f = zeros(4, 1);

    for i = 1:4
        alpha  = alpha_vec(i);
        beta   = beta_vec(i);
        lambda = lambda_vec(i);
        CK     = CK_vec(i);

        % H_accel diagonal + H_yaw diagonal contribution, before final factor of 2
        ele(i) = (beta / ((r * CK)^2)) + lambda + (w * ht^2) / (r^2);

        T_i_prev = T_prev(i);
        K_i_meas = K_meas(i);

        % f_accel term
        % term1 = -alpha * (1 / (r * CK)); % this was original equation
        term1 = -alpha * (CK / r);

        term2_1 = (2 * ((K_i_meas) - (K_opt))) / (r * CK);
        term2_2 = (-2 * (T_i_prev)) / ((r * CK)^2);
        term2 = beta * (term2_1 + term2_2);

        term3 = -2 *lambda * T_i_prev;

        f(i) = term1 + term2 + term3;
    end
    
    % f_yaw contribution
    f(1) = f(1) + Mz_des * (2 * w * ht) / r;
    f(2) = f(2) - Mz_des * (2 * w * ht) / r;
    f(3) = f(3) + Mz_des * (2 * w * ht) / r;
    f(4) = f(4) - Mz_des * (2 * w * ht) / r;

    H = diag(ele) .* 2;

    % Upper off-diagonal
    H12 = (-2 * w * ht^2) / (r^2);
    H13 = (2 * w * ht^2) / (r^2);
    H14 = H12;
    H23 = H12;
    H24 = H13;
    H34 = H12;

    % Lower off-diagonal
    H21 = H12;
    H31 = H13;
    H32 = H23;
    H41 = H14;
    H42 = H24;
    H43 = H34;

    H(1, 2) = H12;
    H(1, 3) = H13;
    H(1, 4) = H14;
    H(2, 1) = H21;
    H(2, 3) = H23;
    H(2, 4) = H24;
    H(3, 1) = H31;
    H(3, 2) = H32;
    H(3, 4) = H34;
    H(4, 1) = H41;
    H(4, 2) = H42;
    H(4, 3) = H43;


    % =========================================================================
    % Power row
    % =========================================================================
    A_power = zeros(1,4);
    for i = 1:4
        eff_i = max(abs(global_eff_vec(i)), 1e-6);
        A_power(i) = (motor_rpm_vec(i) * rpm2rad_s / eff_i) / 11.83;
    end

    Mz_modifier = sign(Mz_des);

    % A_ine = zeros(1, 4);

    % for i = 1:4
    %     A_ine(i) = (motor_rpm_vec(i) * rpm2rad_s / global_eff_vec(i)) / 11.83;
    % end

    % =========================================================================
    % Constraints
    % =========================================================================
    if intent ~= 0

        A_ine = [A_power; % total power
                 diag(A_power); % individual motor power
                 [1 1 1 1]; % total wheel torque
                 diag([1 1 1 1])]; % individual wheel saturation torque
    
        if intent < 0
            A_ine = A_ine .* -1;
        end
    

        A_ine = [A_ine;  
            [-ht/r ht/r -ht/r ht/r] .* Mz_modifier; % desired moment
            [1 -1 0 0]; % FL - FR delta 
            [-1 1 0 0]; % -FL + FR delta
            [0 0 1 -1]; % RL - RR delta 
            [0 0 -1 1]; % -RL + RR delta
            [1 0 -1 0]; % FL - RL delta 
            [-1 0 1 0]; % -FL + RL delta
            [0 1 0 -1]; % FR - RR delta 
            [0 -1 0 1]; % -FR + RR delta
            ]; 

        b_ine = [elec_powerlimit_kW * 1000;
                    [intent_per_motor_elec_p_lim_kW; intent_per_motor_elec_p_lim_kW; intent_per_motor_elec_p_lim_kW; intent_per_motor_elec_p_lim_kW] .* 1000;
                    tot_wheel_torq;
                    wheel_torq_sat_vec;
                    abs(Mz_des);
                    torq_side_delta * 11.83;
                    torq_side_delta * 11.83;
                    torq_side_delta * 11.83;
                    torq_side_delta * 11.83;
                    torq_long_delta * 11.83;
                    torq_long_delta * 11.83;
                    torq_long_delta * 11.83;
                    torq_long_delta * 11.83;
                    ];

        A_eq = [0 0 0 0];
        b_eq = 0;

    else

        % Mz_modifier = sign(Mz_des);

        A_ine = [A_power; % total power
                 diag(A_power); % individual motor power
                 [1 1 1 1]; % total wheel torque
                 diag([1 1 1 1]); % individual wheel saturation torque
                 [-ht/r ht/r -ht/r ht/r] .* Mz_modifier; % desired moment
                 [1 -1 0 0]; % FL - FR delta 
                 [-1 1 0 0]; % -FL + FR delta
                 [0 0 1 -1]; % RL - RR delta 
                 [0 0 -1 1];  % -RL + RR delta
                 [1 0 -1 0]; % FL - RL delta 
                 [-1 0 1 0]; % -FL + RL delta
                 [0 1 0 -1]; % FR - RR delta 
                 [0 -1 0 1];  % -FR + RR delta
                 ]; 
    
        b_ine = [elec_powerlimit_kW * 1000;
                    [intent_per_motor_elec_p_lim_kW; intent_per_motor_elec_p_lim_kW; intent_per_motor_elec_p_lim_kW; intent_per_motor_elec_p_lim_kW] .* 1000;
                    tot_wheel_torq;
                    wheel_torq_sat_vec;
                    abs(Mz_des);
                    torq_side_delta * 11.83;
                    torq_side_delta * 11.83;
                    torq_side_delta * 11.83;
                    torq_side_delta * 11.83;
                    0 * 11.83;
                    0 * 11.83;
                    0 * 11.83;
                    0 * 11.83;
                    ];
    

        A_eq = [1 1 1 1];
        b_eq = tot_wheel_torq;

        if vx_m_s < 2 || abs(Mz_des) < 5
            ub = ub .* 0;
            lb = lb .* 0;
        end

    end
    % x0 = [0; 0; 0; 0];
    opts = optimoptions("quadprog", Algorithm="active-set");

    if intent ~= 0

        lb = min(lb, ub);
        % lb(1) = min(lb(1), ub(1));
        % lb(2) = min(lb(2), ub(2));
        % lb(3) = min(lb(3), ub(3));
        % lb(4) = min(lb(4), ub(4));

        wheel_torque = quadprog(H, f, A_ine, b_ine, [], [], lb, ub, T_prev, opts);
    else

        ub = max(lb, ub);
        % ub(1) = max(lb(1), ub(1));
        % ub(2) = max(lb(2), ub(2));
        % ub(3) = max(lb(3), ub(3));
        % ub(4) = max(lb(4), ub(4));

        wheel_torque = quadprog(H, f, A_ine, b_ine, A_eq, b_eq, lb, ub, T_prev, opts);
    end

    if isempty(wheel_torque)
        wheel_torque   = zeros(4,1);
        elec_theo_p_kW = 0;
        Mz_add         = 0;
        return;
    end

    elec_theo_p_kW = (A_power(1, :) * wheel_torque) / 1000;

    if intent < 0
        elec_theo_p_kW = -abs(elec_theo_p_kW);
    end

    Mz_add = [-ht/r ht/r -ht/r ht/r] * wheel_torque;

== matlab function qp_torq_allocator_base/MATLAB Function1 ==
  data: amk_elec_p_kW_tot input; intent_elec_powerlimit_kW input; w output; w_starting input; w_ending input; w_derate_starting_kW_delta input; w_derate_ending_kW_delta input
function w = fcn(amk_elec_p_kW_tot, intent_elec_powerlimit_kW, w_starting, w_ending, w_derate_starting_kW_delta, w_derate_ending_kW_delta)

amk_elec_p_kW_tot = abs(amk_elec_p_kW_tot);
power_lb = abs(intent_elec_powerlimit_kW) - abs(w_derate_starting_kW_delta);
power_ub = abs(intent_elec_powerlimit_kW) - abs(w_derate_ending_kW_delta);

if power_lb < 0
    power_lb = 0;
end

if power_ub < 0
    power_ub = 0;
end

if power_lb == power_ub
    w = w_ending;
else
    
    if amk_elec_p_kW_tot >= power_lb

        if amk_elec_p_kW_tot > power_ub
            amk_elec_p_kW_tot = 75;
        end

        w = interp1([power_lb power_ub], [w_starting, w_ending], amk_elec_p_kW_tot);
    else
        w = w_starting;
    end

end

== matlab function qp_torq_allocator_base/MATLAB Function2 ==
  data: w_starting input; w_ending input; w_derate output; intent input; use_intent_w_derate input
function w_derate = fcn(w_starting, w_ending, intent, use_intent_w_derate)

if use_intent_w_derate

    if (intent) >= 0.9
        w_derate = interp1([0.9 1], [w_starting, w_ending], (intent));
    else
        w_derate = w_starting;
    end

else

    w_derate = w_starting;
    
end

== matlab function qp_torq_allocator_base/MATLAB Function3 ==
  data: motor_overload_vec input; overload_torq_lim_fl output; overload_derate_x1 input; overload_derate_x2 input; overload_derate_y1 input; overload_derate_y2 input; overload_torq_lim_fr output; overload_torq_lim_rl output; overload_torq_lim_rr output; overload_derate_flag_fl output; overload_derate_flag_fr output; overload_derate_flag_rl output; overload_derate_flag_rr output
function  [overload_torq_lim_fl, overload_torq_lim_fr, overload_torq_lim_rl, overload_torq_lim_rr, overload_derate_flag_fl, overload_derate_flag_fr, overload_derate_flag_rl, overload_derate_flag_rr] = fcn(motor_overload_vec, overload_derate_x1, overload_derate_x2, overload_derate_y1, overload_derate_y2)

overload_torq_lim = zeros(4, 1);
overload_derate_flag = zeros(4, 1);

for i = 1:length(motor_overload_vec)
    if motor_overload_vec(i) > overload_derate_x2
        motor_overload_vec(i) = overload_derate_x2;
    end

    if motor_overload_vec(i) < overload_derate_x1
        motor_overload_vec(i) = overload_derate_x1;
    end

    overload_torq_lim(i) = interp1([overload_derate_x1, overload_derate_x2], [overload_derate_y1, overload_derate_y2], motor_overload_vec(i));
    
    if overload_torq_lim(i) < overload_derate_y1
        overload_derate_flag(i) = 1;
    end
end

overload_torq_lim_fl = overload_torq_lim(1);
overload_torq_lim_fr = overload_torq_lim(2);
overload_torq_lim_rl = overload_torq_lim(3);
overload_torq_lim_rr = overload_torq_lim(4);

overload_derate_flag_fl = overload_derate_flag(1);
overload_derate_flag_fr = overload_derate_flag(2);
overload_derate_flag_rl = overload_derate_flag(3);
overload_derate_flag_rr = overload_derate_flag(4);
